simulink model "top_model"  (R2018a)
settings: Solver=FixedStepAuto  StartTime=0.0  StopTime=600  FixedStep=.01  RelTol=1e-3  EnableMultiTasking=on
model workspace: external: MAT-File C:\Users\Justin\Documents\00 MEng Project\PAN_ADCS\initialization\simulink_workspace_init.mat (data not in the file)
undefined symbols (not defined in the file or in its folder): h_init, hdmax, hmax, IAU, Imp_max, Imp_min, init, K_F, Kd, km, Kp, L_F, m_follower, match_tol, muE, ontime_max, ontime_min, q_init, s, Thrust_max, Thrust_min, wbn_init
libraries: aerolibtransform2 x9, hEemethod x8, aerolibconvert2 x6, aerolibgravity2 x5, sharedtransform x4, aerolibutil x4, aerolibcelestial x3, vrlib x2
(part 2 of 3)

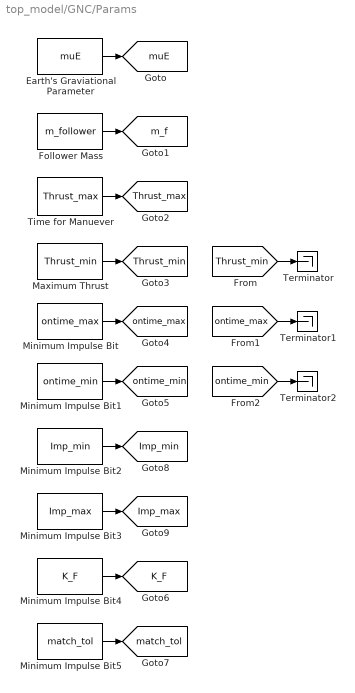
== system top_model/GNC/Params ==
  Earth's Graviational Parameter : Constant  Value=muE
  Follower Mass : Constant  Value=m_follower
  Maximum Thrust : Constant  Value=Thrust_min
  Minimum Impulse Bit : Constant  Value=ontime_max
  Minimum Impulse Bit1 : Constant  Value=ontime_min
  Minimum Impulse Bit2 : Constant  Value=Imp_min
  Minimum Impulse Bit3 : Constant  Value=Imp_max
  Minimum Impulse Bit4 : Constant  Value=K_F
  Minimum Impulse Bit5 : Constant  Value=match_tol
  Terminator : Terminator
  Terminator1 : Terminator
  Terminator2 : Terminator
  Time for Manuever : Constant  Value=Thrust_max
  tag scope: Imp_max=global, Imp_min=global, K_F=global, Thrust_max=global, Thrust_min=global, m_f=global, match_tol=global, muE=global, ontime_max=global, ontime_min=global
  wires:
  Time for Manuever/1 -> [Thrust_max]
  Follower Mass/1 -> [m_f]
  Earth's Graviational Parameter/1 -> [muE]
  Maximum Thrust/1 -> [Thrust_min]
  Minimum Impulse Bit/1 -> [ontime_max]
  Minimum Impulse Bit1/1 -> [ontime_min]
  Minimum Impulse Bit2/1 -> [Imp_min]
  Minimum Impulse Bit3/1 -> [Imp_max]
  [Thrust_min] -> Terminator/1
  [ontime_max] -> Terminator1/1
  [ontime_min] -> Terminator2/1
  Minimum Impulse Bit4/1 -> [K_F]
  Minimum Impulse Bit5/1 -> [match_tol]

== system top_model/LDR_Plant/Cross ==
  A : Inport
  B : Inport  Port=2
  Mux4 : Mux  Inputs=3
  Product{,1..5} (6 alike) : Product  SaturateOnIntegerOverflow=on  InputSameDT=on  OutDataTypeStr=Inherit: Same as first input
  Sum : Sum  Inputs=+-  SaturateOnIntegerOverflow=on  InputSameDT=on  OutDataTypeStr=Inherit: Same as first input
  Sum1 : Sum  Inputs=+-  SaturateOnIntegerOverflow=on  InputSameDT=on  OutDataTypeStr=Inherit: Same as first input
  Sum2 : Sum  Inputs=+-  SaturateOnIntegerOverflow=on  InputSameDT=on  OutDataTypeStr=Inherit: Same as first input
  demux2 : Demux  Outputs=3
  demux3 : Demux  Outputs=3
  AxB : Outport  InitialOutput=0
  wires:
  Mux4/1 -> AxB/1
  Sum2/1 -> Mux4/3
  Sum1/1 -> Mux4/2
  Sum/1 -> Mux4/1
  Product5/1 -> Sum2/2
  Product4/1 -> Sum2/1
  Product3/1 -> Sum1/2
  Product2/1 -> Sum1/1
  Product1/1 -> Sum/2
  Product/1 -> Sum/1
  demux3/1 -> Product5/2, Product2/2
  demux2/2 -> Product5/1, Product/1
  demux3/2 -> Product4/2, Product1/2
  demux2/1 -> Product4/1, Product3/1
  demux3/3 -> Product3/2, Product/2
  demux2/3 -> Product2/1, Product1/1
  B/1 -> demux3/1
  A/1 -> demux2/1

== system top_model/LDR_Plant/DecimalYearIncrement ==
  note: day
  clock_sec : Inport
  Add : Sum
  Constant : Constant  Value=init.year
  Constant1 : Constant  Value=init.month
  Constant2 : Constant  Value=init.day
  Constant3 : Constant  Value=init.hour
  Constant4 : Constant  Value=init.min
  Constant5 : Constant  Value=init.min
  Divide : Product  Inputs=*/
  MATLAB Function : MATLAB Function  TreatAsAtomicUnit=on
  Product2 : Product  Inputs=*/
  day2decimalYear : Constant  Value=365
  sec2day : Constant  Value=86400
  DecimalYear : Outport
  wires:
  Product2/1 -> Divide/1
  sec2day/1 -> Product2/2
  Add/1 -> DecimalYear/1
  Constant3/1 -> MATLAB Function/4(hour)
  day2decimalYear/1 -> Divide/2
  Divide/1 -> Add/1
  MATLAB Function/1(DecimalYear) -> Add/2
  Constant1/1 -> MATLAB Function/2(month)
  Constant/1 -> MATLAB Function/1(year)
  Constant4/1 -> MATLAB Function/5(minute)
  Constant5/1 -> MATLAB Function/6(second)
  clock_sec/1 -> Product2/1
  Constant2/1 -> MATLAB Function/3(day)

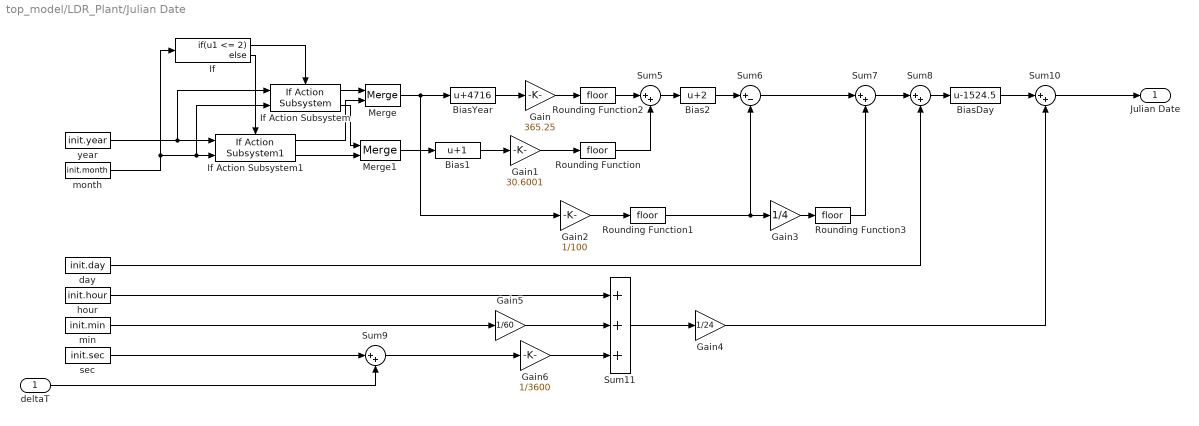
== system top_model/LDR_Plant/Julian Date ==
  deltaT : Inport  OutMin=0  PortDimensions=1
  Bias1 : Bias  Bias=1
  Bias2 : Bias  Bias=2
  BiasDay : Bias  Bias=-1524.5
  BiasYear : Bias  Bias=4716
  Gain : Gain  Gain=365.25
  Gain1 : Gain  Gain=30.6001
  Gain2 : Gain  Gain=1/100
  Gain3 : Gain  Gain=1/4
  Gain4 : Gain  Gain=1/24
  Gain5 : Gain  Gain=1/60
  Gain6 : Gain  Gain=1/3600
  If : If  IfExpression=u1 <= 2
  If Action Subsystem : aerolibconvert2/Julian Date Conversion/If Action Subsystem
      settings: SourceProductName=Aerospace Blockset  SourceProductBaseCode=AE
  If Action Subsystem1 : aerolibconvert2/Julian Date Conversion/If Action Subsystem1
      settings: SourceProductName=Aerospace Blockset  SourceProductBaseCode=AE
  Merge : Merge
  Merge1 : Merge
  Rounding Function{,1..3} (4 alike) : Rounding
  Sum{5,7..10} (5 alike) : Sum  Inputs=|++
  Sum11 : Sum  Inputs=+++
  Sum6 : Sum  Inputs=|+-
  day : Constant  Value=init.day
  hour : Constant  Value=init.hour
  min : Constant  Value=init.min
  month : Constant  Value=init.month
  sec : Constant  Value=init.sec
  year : Constant  Value=init.year
  Julian Date : Outport
  wires:
  If Action Subsystem/1 -> Merge/1
  If/2 -> If Action Subsystem1/Action
  year/1 -> If Action Subsystem/1, If Action Subsystem1/1
  If/1 -> If Action Subsystem/Action
  If Action Subsystem/2 -> Merge1/1
  Rounding Function3/1 -> Sum7/2
  deltaT/1 -> Sum9/2
  Merge1/1 -> Bias1/1
  Gain/1 -> Rounding Function2/1
  Gain2/1 -> Rounding Function1/1
  Merge/1 -> Gain2/1, BiasYear/1
  Sum9/1 -> Gain6/1
  Sum6/1 -> Sum7/1
  Gain5/1 -> Sum11/2
  BiasYear/1 -> Gain/1
  min/1 -> Gain5/1
  Gain6/1 -> Sum11/3
  Sum11/1 -> Gain4/1
  Gain3/1 -> Rounding Function3/1
  hour/1 -> Sum11/1
  If Action Subsystem1/1 -> Merge/2
  Sum7/1 -> Sum8/1
  Sum10/1 -> Julian Date/1
  day/1 -> Sum8/2
  Bias1/1 -> Gain1/1
  sec/1 -> Sum9/1
  If Action Subsystem1/2 -> Merge1/2
  Sum5/1 -> Bias2/1
  BiasDay/1 -> Sum10/1
  Gain1/1 -> Rounding Function/1
  Rounding Function1/1 -> Gain3/1, Sum6/2
  Bias2/1 -> Sum6/1
  Sum8/1 -> BiasDay/1
  Rounding Function2/1 -> Sum5/1
  Rounding Function/1 -> Sum5/2
  month/1 -> If Action Subsystem/2, If Action Subsystem1/2, If/1
  Gain4/1 -> Sum10/2

== system top_model/LDR_Plant/Quaternion Integration ==
  w_Body : Inport
  Gain : Gain  Gain=-1
  Integrator1 : Integrator  InitialCondition=init.LDR.q_init  ContinuousStateAttributes='quaternion_plant'
  Selector : Selector  InputPortWidth=4  IndexOptions=Index vector (dialog)  Indices=4  OutputSizes=1
  Switch : Switch  Criteria=u2 > Threshold
  q_normalize : Subsystem
  qderiv : Subsystem
  q_I_Body : Outport
  wires:
  qderiv/1(qd) -> Integrator1/1
  Integrator1/1 -> q_normalize/1(q_in)
  q_normalize/1(q_out) -> Gain/1, Selector/1, q_I_Body/1, Switch/1, qderiv/2(q)
  w_Body/1 -> qderiv/1(w)
  Selector/1 -> Switch/2
  Gain/1 -> Switch/3

== system top_model/LDR_Sensor Model/Magnetometer ==
  note: Magnetometer: LIS3MDL
      | see the data sheet for more details
  Magnetic_Field_body : Inport  Unit=nT
  DCM to translate from body to sensor : Constant  Value=init.IMU0_DCM_BODY
  Data Type Conversion : DataTypeConversion  OutDataTypeStr=int16  RndMeth=Round
  Matrix Multiply2 : Product  Multiplication=Matrix(*)
  Random Number : RandomNumber  Mean=-init.IMU0_ZGAUSS  Variance=init.IMU0_RMS^2  SampleTime=1.0/init.IMU0_MAG_ODR
  Sum : Sum  Inputs=|++
  Zero-Order Hold : ZeroOrderHold  SampleTime=1.0/init.IMU0_MAG_ODR
  nT to gauss : Gain  Gain=1.0e-5
  sensitivity : Gain  Gain=init.IMU0_MAG_GN
  Magxyz : Outport  OutDataTypeStr=int16
  wires:
  Data Type Conversion/1 -> Magxyz/1
  sensitivity/1 -> Data Type Conversion/1
  nT to gauss/1 -> Zero-Order Hold/1
  Zero-Order Hold/1 -> Sum/1
  Sum/1 -> sensitivity/1
  Random Number/1 -> Sum/2
  Matrix Multiply2/1 -> nT to gauss/1
  Magnetic_Field_body/1 -> Matrix Multiply2/2
  DCM to translate from body to sensor/1 -> Matrix Multiply2/1

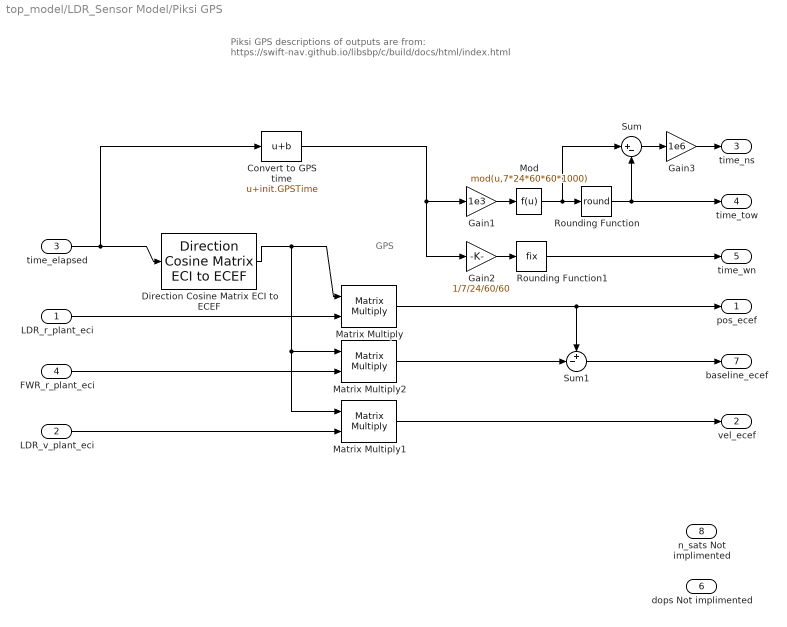
== system top_model/LDR_Sensor Model/Piksi GPS ==
  note: Piksi GPS
      |
      | descriptions of outputs are from:
      | https://swift-nav.github.io/libsbp/c/build/docs/html/index.html
  note: GPS
  LDR_r_plant_eci : Inport
  LDR_v_plant_eci : Inport  Port=2
  time_elapsed : Inport  Port=3
  FWR_r_plant_eci : Inport  Port=4
  Convert to GPS time : Bias  Bias=init.GPSTime
  Direction Cosine Matrix ECI to ECEF : aerolibtransform2/Direction Cosine Matrix ECI to ECEF  red=IAU-2000/2006  year=init.year  month=October  day=20  hour=init.hour  min=init.min  sec=init.sec  deltaT=Sec  errorflag=Error  extraparamflag=off
      settings: AttributesFormatString=%<red>  SourceProductName=Aerospace Blockset  SourceProductBaseCode=AE
  Gain1 : Gain  Gain=1e3
  Gain2 : Gain  Gain=1/7/24/60/60
  Gain3 : Gain  Gain=1e6
  Matrix Multiply : Product  Multiplication=Matrix(*)
  Matrix Multiply1 : Product  Multiplication=Matrix(*)
  Matrix Multiply2 : Product  Multiplication=Matrix(*)
  Mod : Fcn  Expr=mod(u,7*24*60*60*1000)
  Rounding Function : Rounding  Operator=round
  Rounding Function1 : Rounding  Operator=fix
  Sum : Sum  Inputs=|+-
  Sum1 : Sum  Inputs=+-|
  pos_ecef : Outport  OutDataTypeStr=double  Unit=m
      settings: AttributesFormatString=absolute Earth Centered Earth Fixed (ECEF) coordinates
  vel_ecef : Outport  Port=2  OutDataTypeStr=int32  Unit=mm/s
      settings: AttributesFormatString=velocity in Earth Centered Earth Fixed (ECEF) coordinates.
  time_ns : Outport  Port=3  OutMin=[-500000]  OutMax=[500000]  OutDataTypeStr=int32  Unit=ns
      settings: AttributesFormatString=Nanosecond residual of millisecond-rounded TOW
  time_tow : Outport  Port=4  OutMin=[0]  OutDataTypeStr=uint32  Unit=ms
      settings: AttributesFormatString=GPS time of week rounded to the nearest millisecond
  time_wn : Outport  Port=5  OutDataTypeStr=uint16  Unit=weeks
      settings: AttributesFormatString=GPS week number
  dops Not implimented : Outport  Port=6
      settings: AttributesFormatString=|
      | Dilution of Precision p,t
      | describes the effect of navigation satellite geometry on positional measurement precision.
  baseline_ecef : Outport  Description=Dilution of Precision p,t  Port=7  OutDataTypeStr=int32  Unit=mm
      settings: AttributesFormatString=relative vector distance from the base station to the rover receiver.
  n_sats Not implimented : Outport  Port=8  OutDataTypeStr=uint8
      settings: AttributesFormatString=Number of satellites used in solution.
  wires:
  Direction Cosine Matrix ECI to ECEF/1 -> Matrix Multiply1/1, Matrix Multiply2/1, Matrix Multiply/1
  time_elapsed/1 -> Convert to GPS time/1, Direction Cosine Matrix ECI to ECEF/1
  LDR_v_plant_eci/1 -> Matrix Multiply1/2
  Matrix Multiply1/1 -> vel_ecef/1
  Matrix Multiply/1 -> Sum1/1, pos_ecef/1
  LDR_r_plant_eci/1 -> Matrix Multiply/2
  Convert to GPS time/1 -> Gain2/1, Gain1/1
  Gain2/1 -> Rounding Function1/1
  Rounding Function1/1 -> time_wn/1
  Gain1/1 -> Mod/1
  Mod/1 -> Sum/1, Rounding Function/1
  Rounding Function/1 -> Sum/2, time_tow/1
  Sum/1 -> Gain3/1
  Gain3/1 -> time_ns/1
  FWR_r_plant_eci/1 -> Matrix Multiply2/2
  Sum1/1 -> baseline_ecef/1
  Matrix Multiply2/1 -> Sum1/2

== system top_model/LDR_Sensor Model/quat to DCM ==
  e0 e1 e2 e3 : Inport
  Demux : Demux
  Gain1 : Gain  Gain=2  SaturateOnIntegerOverflow=on  OutDataTypeStr=Inherit: Same as input  ParamDataTypeStr=Inherit: Same as input
  Gain2 : Gain  Gain=2  SaturateOnIntegerOverflow=on  OutDataTypeStr=Inherit: Same as input  ParamDataTypeStr=Inherit: Same as input
  Matrix Gain : Gain  Gain=eye(3,3)  SaturateOnIntegerOverflow=on  OutDataTypeStr=Inherit: Same as input  ParamDataTypeStr=Inherit: Same as input
  Mux : Mux  Inputs=3
  Product : Product  SaturateOnIntegerOverflow=on  InputSameDT=on  OutDataTypeStr=Inherit: Same as first input
  Product1 : Product  SaturateOnIntegerOverflow=on  InputSameDT=on  OutDataTypeStr=Inherit: Same as first input
  Subsystem : Subsystem
      mask Display: disp('3x3 cross matrix')
  Sum1 : Sum  Inputs=|+-  SaturateOnIntegerOverflow=on  InputSameDT=on  OutDataTypeStr=Inherit: Same as first input
  Sum8 : Sum  Inputs=|+-+  SaturateOnIntegerOverflow=on  InputSameDT=on  OutDataTypeStr=Inherit: Same as first input
  T1 : Math  Operator=transpose  SaturateOnIntegerOverflow=on
  T2 : Math  Operator=transpose  SaturateOnIntegerOverflow=on
  qTq : Product  Multiplication=Matrix(*)  SaturateOnIntegerOverflow=on  InputSameDT=on  OutDataTypeStr=Inherit: Same as first input
  qqT : Product  Multiplication=Matrix(*)  SaturateOnIntegerOverflow=on  InputSameDT=on  OutDataTypeStr=Inherit: Same as first input
  DCM : Outport  InitialOutput=0
  wires:
  Sum8/1 -> DCM/1
  e0 e1 e2 e3/1 -> Demux/1
  Demux/1 -> Mux/1
  Demux/2 -> Mux/2
  Demux/3 -> Mux/3
  Demux/4 -> Product/2, Product1/1, Product1/2
  Mux/1 -> T1/1, qqT/1, Subsystem/1(In1), T2/1, qTq/2
  Product/1 -> Gain1/1
  T1/1 -> qqT/2
  qqT/1 -> Gain2/1
  Gain2/1 -> Sum8/1
  Gain1/1 -> Sum8/2
  Product1/1 -> Sum1/1
  T2/1 -> qTq/1
  qTq/1 -> Sum1/2
  Sum1/1 -> Matrix Gain/1
  Matrix Gain/1 -> Sum8/3
  Subsystem/1(Out1) -> Product/1

== system top_model/Actuator Model/Rigid Body with Momentum Actuators and energy dissipation/Cross1 ==
  A : Inport  PortDimensions=3
  B : Inport  Port=2  PortDimensions=3
  Mux4 : Mux  Inputs=3
  Product{,1..5} (6 alike) : Product  SaturateOnIntegerOverflow=on  InputSameDT=on  OutDataTypeStr=Inherit: Same as first input
  Sum : Sum  Inputs=+-  SaturateOnIntegerOverflow=on  InputSameDT=on  OutDataTypeStr=Inherit: Same as first input
  Sum1 : Sum  Inputs=+-  SaturateOnIntegerOverflow=on  InputSameDT=on  OutDataTypeStr=Inherit: Same as first input
  Sum2 : Sum  Inputs=+-  SaturateOnIntegerOverflow=on  InputSameDT=on  OutDataTypeStr=Inherit: Same as first input
  demux2 : Demux  Outputs=3
  demux3 : Demux  Outputs=3
  AxB : Outport  InitialOutput=0
  wires:
  Mux4/1 -> AxB/1
  Sum2/1 -> Mux4/3
  Sum1/1 -> Mux4/2
  Sum/1 -> Mux4/1
  Product5/1 -> Sum2/2
  Product4/1 -> Sum2/1
  Product3/1 -> Sum1/2
  Product2/1 -> Sum1/1
  Product1/1 -> Sum/2
  Product/1 -> Sum/1
  demux3/1 -> Product5/2, Product2/2
  demux2/2 -> Product5/1, Product/1
  demux3/2 -> Product4/2, Product1/2
  demux2/1 -> Product4/1, Product3/1
  demux3/3 -> Product3/2, Product/2
  demux2/3 -> Product2/1, Product1/1
  B/1 -> demux3/1
  A/1 -> demux2/1

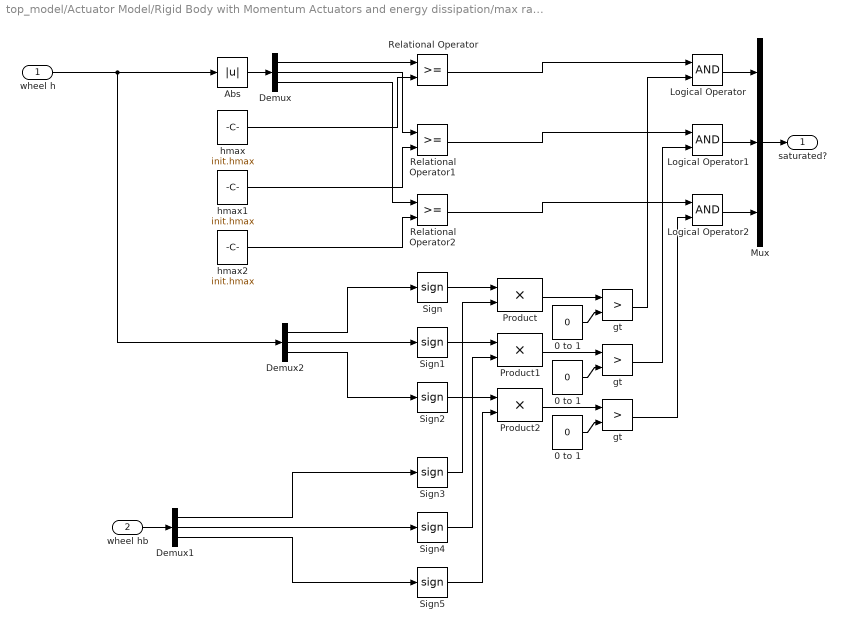
== system top_model/Actuator Model/Rigid Body with Momentum Actuators and energy dissipation/max rate check ==
  wheel h : Inport
  wheel hb : Inport  Port=2
  0 to 1 : Constant  Value=0  VectorParams1D=off
  "0 to 1 " : Constant  Value=0  VectorParams1D=off
  "0 to 1  " : Constant  Value=0  VectorParams1D=off
  Abs : Abs  SaturateOnIntegerOverflow=on
  Demux : Demux  Outputs=3
  Demux1 : Demux  Outputs=3
  Demux2 : Demux  Outputs=3
  Logical Operator : Logic
  Logical Operator1 : Logic
  Logical Operator2 : Logic
  Mux : Mux  Inputs=3
  Product : Product  SaturateOnIntegerOverflow=on  InputSameDT=on  OutDataTypeStr=Inherit: Same as first input
  Product1 : Product  SaturateOnIntegerOverflow=on  InputSameDT=on  OutDataTypeStr=Inherit: Same as first input
  Product2 : Product  SaturateOnIntegerOverflow=on  InputSameDT=on  OutDataTypeStr=Inherit: Same as first input
  Relational Operator : RelationalOperator  RndMeth=Nearest  InputSameDT=on
  Relational Operator1 : RelationalOperator  RndMeth=Nearest  InputSameDT=on
  Relational Operator2 : RelationalOperator  RndMeth=Nearest  InputSameDT=on
  Sign{,1..5} (6 alike) : Signum
  gt : RelationalOperator  Operator=>  RndMeth=Nearest  InputSameDT=on
  "gt " : RelationalOperator  Operator=>  RndMeth=Nearest  InputSameDT=on
  "gt  " : RelationalOperator  Operator=>  RndMeth=Nearest  InputSameDT=on
  hmax : Constant  Value=init.hmax  VectorParams1D=off
  hmax1 : Constant  Value=init.hmax  VectorParams1D=off
  hmax2 : Constant  Value=init.hmax  VectorParams1D=off
  saturated? : Outport
  wires:
  Abs/1 -> Demux/1
  Demux/1 -> Relational Operator/1
  Demux/2 -> Relational Operator1/1
  Demux/3 -> Relational Operator2/1
  hmax/1 -> Relational Operator/2
  hmax1/1 -> Relational Operator1/2
  hmax2/1 -> Relational Operator2/2
  wheel h/1 -> Abs/1, Demux2/1
  Mux/1 -> saturated?/1
  wheel hb/1 -> Demux1/1
  Demux1/1 -> Sign3/1
  Demux1/2 -> Sign4/1
  Demux1/3 -> Sign5/1
  Sign/1 -> Product/1
  Sign3/1 -> Product/2
  Sign1/1 -> Product1/1
  Sign4/1 -> Product1/2
  Sign2/1 -> Product2/1
  Sign5/1 -> Product2/2
  0 to 1/1 -> gt/2
  Product/1 -> gt/1
  "0 to 1 "/1 -> "gt "/2
  Product1/1 -> "gt "/1
  "0 to 1  "/1 -> "gt  "/2
  Product2/1 -> "gt  "/1
  Logical Operator/1 -> Mux/1
  Logical Operator1/1 -> Mux/2
  Logical Operator2/1 -> Mux/3
  Relational Operator/1 -> Logical Operator/1
  Relational Operator1/1 -> Logical Operator1/1
  Relational Operator2/1 -> Logical Operator2/1
  gt/1 -> Logical Operator/2
  "gt "/1 -> Logical Operator1/2
  "gt  "/1 -> Logical Operator2/2
  Demux2/1 -> Sign/1
  Demux2/2 -> Sign1/1
  Demux2/3 -> Sign2/1

== system top_model/Actuator Model/Rigid Body with Momentum Actuators and energy dissipation/quat to DCM ==
  e0 e1 e2 e3 : Inport
  Demux : Demux
  Gain1 : Gain  Gain=2  SaturateOnIntegerOverflow=on  OutDataTypeStr=Inherit: Same as input  ParamDataTypeStr=Inherit: Same as input
  Gain2 : Gain  Gain=2  SaturateOnIntegerOverflow=on  OutDataTypeStr=Inherit: Same as input  ParamDataTypeStr=Inherit: Same as input
  Matrix Gain : Gain  Gain=eye(3,3)  SaturateOnIntegerOverflow=on  OutDataTypeStr=Inherit: Same as input  ParamDataTypeStr=Inherit: Same as input
  Mux : Mux  Inputs=3
  Product : Product  SaturateOnIntegerOverflow=on  InputSameDT=on  OutDataTypeStr=Inherit: Same as first input
  Product1 : Product  SaturateOnIntegerOverflow=on  InputSameDT=on  OutDataTypeStr=Inherit: Same as first input
  Subsystem : Subsystem
      mask Display: disp('3x3 cross matrix')
  Sum1 : Sum  Inputs=|+-  SaturateOnIntegerOverflow=on  InputSameDT=on  OutDataTypeStr=Inherit: Same as first input
  Sum8 : Sum  Inputs=|+-+  SaturateOnIntegerOverflow=on  InputSameDT=on  OutDataTypeStr=Inherit: Same as first input
  T1 : Math  Operator=transpose  SaturateOnIntegerOverflow=on
  T2 : Math  Operator=transpose  SaturateOnIntegerOverflow=on
  qTq : Product  Multiplication=Matrix(*)  SaturateOnIntegerOverflow=on  InputSameDT=on  OutDataTypeStr=Inherit: Same as first input
  qqT : Product  Multiplication=Matrix(*)  SaturateOnIntegerOverflow=on  InputSameDT=on  OutDataTypeStr=Inherit: Same as first input
  DCM : Outport  InitialOutput=0
  wires:
  Subsystem/1(Out1) -> Product/1
  Matrix Gain/1 -> Sum8/3
  Sum1/1 -> Matrix Gain/1
  qTq/1 -> Sum1/2
  T2/1 -> qTq/1
  Product1/1 -> Sum1/1
  Gain1/1 -> Sum8/2
  Gain2/1 -> Sum8/1
  qqT/1 -> Gain2/1
  T1/1 -> qqT/2
  Product/1 -> Gain1/1
  Mux/1 -> qTq/2, T2/1, qqT/1, T1/1, Subsystem/1(In1)
  Demux/4 -> Product1/2, Product1/1, Product/2
  Demux/3 -> Mux/3
  Demux/2 -> Mux/2
  Demux/1 -> Mux/1
  e0 e1 e2 e3/1 -> Demux/1
  Sum8/1 -> DCM/1

== system top_model/Actuator Model/Rigid Body with Momentum Actuators and energy dissipation/quat to DCM1 ==
  e0 e1 e2 e3 : Inport
  Demux : Demux
  Gain1 : Gain  Gain=2  SaturateOnIntegerOverflow=on  OutDataTypeStr=Inherit: Same as input  ParamDataTypeStr=Inherit: Same as input
  Gain2 : Gain  Gain=2  SaturateOnIntegerOverflow=on  OutDataTypeStr=Inherit: Same as input  ParamDataTypeStr=Inherit: Same as input
  Matrix Gain : Gain  Gain=eye(3,3)  SaturateOnIntegerOverflow=on  OutDataTypeStr=Inherit: Same as input  ParamDataTypeStr=Inherit: Same as input
  Mux : Mux  Inputs=3
  Product : Product  SaturateOnIntegerOverflow=on  InputSameDT=on  OutDataTypeStr=Inherit: Same as first input
  Product1 : Product  SaturateOnIntegerOverflow=on  InputSameDT=on  OutDataTypeStr=Inherit: Same as first input
  Subsystem : Subsystem
      mask Display: disp('3x3 cross matrix')
  Sum1 : Sum  Inputs=|+-  SaturateOnIntegerOverflow=on  InputSameDT=on  OutDataTypeStr=Inherit: Same as first input
  Sum8 : Sum  Inputs=|+-+  SaturateOnIntegerOverflow=on  InputSameDT=on  OutDataTypeStr=Inherit: Same as first input
  T1 : Math  Operator=transpose  SaturateOnIntegerOverflow=on
  T2 : Math  Operator=transpose  SaturateOnIntegerOverflow=on
  qTq : Product  Multiplication=Matrix(*)  SaturateOnIntegerOverflow=on  InputSameDT=on  OutDataTypeStr=Inherit: Same as first input
  qqT : Product  Multiplication=Matrix(*)  SaturateOnIntegerOverflow=on  InputSameDT=on  OutDataTypeStr=Inherit: Same as first input
  DCM : Outport  InitialOutput=0
  wires:
  Subsystem/1(Out1) -> Product/1
  Matrix Gain/1 -> Sum8/3
  Sum1/1 -> Matrix Gain/1
  qTq/1 -> Sum1/2
  T2/1 -> qTq/1
  Product1/1 -> Sum1/1
  Gain1/1 -> Sum8/2
  Gain2/1 -> Sum8/1
  qqT/1 -> Gain2/1
  T1/1 -> qqT/2
  Product/1 -> Gain1/1
  Mux/1 -> qTq/2, T2/1, qqT/1, T1/1, Subsystem/1(In1)
  Demux/4 -> Product1/2, Product1/1, Product/2
  Demux/3 -> Mux/3
  Demux/2 -> Mux/2
  Demux/1 -> Mux/1
  e0 e1 e2 e3/1 -> Demux/1
  Sum8/1 -> DCM/1

== system top_model/Attitude Determination and Desired Attitude/Attitude Determination/Generate reference vectors from Ephemeris and Magnetic Field Model ==
  note: geodetic LLA
  time_elapsed : Inport
  r_cs_sensor_eci : Inport  Port=2
  Add : Sum  Inputs=+-
  DecimalYearIncrement : Subsystem
  Demux : Demux  Outputs=3
  ECI Position to LLA : aerolibtransform2/ECI Position to LLA  red=IAU-2000/2006  year=init.year  month=October  day=20  hour=init.hour  min=init.min  sec=init.sec  deltaT=Sec  errorflag=Error  extraparamflag=off  eunits=Metric (MKS)  earthmodel=WGS84  flat=1/298.257223563  eqradius=6378137
      settings: AttributesFormatString=%<red>  SourceProductName=Aerospace Blockset  SourceProductBaseCode=AE
  International Geomagnetic Reference Field 12 : aerolibgravity2/International Geomagnetic Reference Field 12  units=Metric (MKS)  time_in=on  month=January  day=1  year=2020  action=None  sv_out=off
      settings: SourceProductName=Aerospace Blockset  SourceProductBaseCode=AE
  Julian Date : Subsystem
  Planetary Ephemeris : aerolibcelestial/Planetary Ephemeris  kmflag=km,km/s  epochflag=Julian date  de=DE430  nCenter=Earth  nTarget=Sun  errorflag=Error  velflag=off
      settings: SourceProductName=Aerospace Blockset  SourceProductBaseCode=AE
  r_Sun2cs_ref_eci : Outport
  r_MagField_ref_eci : Outport  Port=2
  wires:
  Julian Date/1(Julian Date) -> Planetary Ephemeris/1
  Planetary Ephemeris/1 -> Add/1
  Demux/1 -> International Geomagnetic Reference Field 12/2
  International Geomagnetic Reference Field 12/1 -> r_MagField_ref_eci/1
  ECI Position to LLA/1 -> Demux/1
  Demux/3 -> International Geomagnetic Reference Field 12/1
  Add/1 -> r_Sun2cs_ref_eci/1
  DecimalYearIncrement/1(DecimalYear) -> International Geomagnetic Reference Field 12/4
  r_cs_sensor_eci/1 -> Add/2, ECI Position to LLA/1
  time_elapsed/1 -> DecimalYearIncrement/1(clock_sec), ECI Position to LLA/2, Julian Date/1(deltaT)
  Demux/2 -> International Geomagnetic Reference Field 12/3

== system top_model/Attitude Determination and Desired Attitude/Attitude Determination/Subsystem ==
  r_Sun2cs_ref_eci : Inport
  r_MagField_ref_eci : Inport  Port=2
  r_Sun2cs_sensor_body : Inport  Port=3
  r_MagField_sensor_body : Inport  Port=4
  MATLAB Function : MATLAB Function  TreatAsAtomicUnit=on
  quat_body_calc : Outport
  wires:
  r_Sun2cs_ref_eci/1 -> MATLAB Function/1(N_sun)
  r_MagField_ref_eci/1 -> MATLAB Function/2(N_mag)
  r_Sun2cs_sensor_body/1 -> MATLAB Function/3(B_sun)
  r_MagField_sensor_body/1 -> MATLAB Function/4(B_mag)
  MATLAB Function/1(q_triad) -> quat_body_calc/1

== system top_model/Attitude Determination and Desired Attitude/Position and Velocity to Desired Attitude in Quat/CreateDCM_be ==
  Position : Inport
  Velocity : Inport  Port=2
  Cross Product : vrlib/Utilities/Cross Product
      settings: SourceProductBaseCode=VR
  Cross Product1 : vrlib/Utilities/Cross Product
      settings: SourceProductBaseCode=VR
  Matrix Concatenate : Concatenate  NumInputs=3  Mode=Multidimensional array  ConcatenateDimension=2
  normalize : Subsystem
  normalize2 : Subsystem
  DCM_be : Outport
  wires:
  normalize/1(r_hat) -> Cross Product1/1, Matrix Concatenate/1
  Cross Product/1 -> normalize2/1(v)
  Velocity/1 -> Cross Product/1
  Matrix Concatenate/1 -> DCM_be/1
  Position/1 -> Cross Product/2, normalize/1(r)
  Cross Product1/1 -> Matrix Concatenate/3
  normalize2/1(v_hat) -> Cross Product1/2, Matrix Concatenate/2

== system top_model/Attitude Determination and Desired Attitude/Position and Velocity to Desired Attitude in Quat/quat to DCM ==
  e0 e1 e2 e3 : Inport
  Demux : Demux
  Gain1 : Gain  Gain=2  SaturateOnIntegerOverflow=on  OutDataTypeStr=Inherit: Same as input  ParamDataTypeStr=Inherit: Same as input
  Gain2 : Gain  Gain=2  SaturateOnIntegerOverflow=on  OutDataTypeStr=Inherit: Same as input  ParamDataTypeStr=Inherit: Same as input
  Matrix Gain : Gain  Gain=eye(3,3)  SaturateOnIntegerOverflow=on  OutDataTypeStr=Inherit: Same as input  ParamDataTypeStr=Inherit: Same as input
  Mux : Mux  Inputs=3
  Product : Product  SaturateOnIntegerOverflow=on  InputSameDT=on  OutDataTypeStr=Inherit: Same as first input
  Product1 : Product  SaturateOnIntegerOverflow=on  InputSameDT=on  OutDataTypeStr=Inherit: Same as first input
  Subsystem : Subsystem
      mask Display: disp('3x3 cross matrix')
  Sum1 : Sum  Inputs=|+-  SaturateOnIntegerOverflow=on  InputSameDT=on  OutDataTypeStr=Inherit: Same as first input
  Sum8 : Sum  Inputs=|+-+  SaturateOnIntegerOverflow=on  InputSameDT=on  OutDataTypeStr=Inherit: Same as first input
  T1 : Math  Operator=transpose  SaturateOnIntegerOverflow=on
  T2 : Math  Operator=transpose  SaturateOnIntegerOverflow=on
  qTq : Product  Multiplication=Matrix(*)  SaturateOnIntegerOverflow=on  InputSameDT=on  OutDataTypeStr=Inherit: Same as first input
  qqT : Product  Multiplication=Matrix(*)  SaturateOnIntegerOverflow=on  InputSameDT=on  OutDataTypeStr=Inherit: Same as first input
  DCM : Outport  InitialOutput=0
  wires:
  Subsystem/1(Out1) -> Product/1
  Matrix Gain/1 -> Sum8/3
  Sum1/1 -> Matrix Gain/1
  qTq/1 -> Sum1/2
  T2/1 -> qTq/1
  Product1/1 -> Sum1/1
  Gain1/1 -> Sum8/2
  Gain2/1 -> Sum8/1
  qqT/1 -> Gain2/1
  T1/1 -> qqT/2
  Product/1 -> Gain1/1
  Mux/1 -> qTq/2, T2/1, qqT/1, T1/1, Subsystem/1(In1)
  Demux/4 -> Product1/2, Product1/1, Product/2
  Demux/3 -> Mux/3
  Demux/2 -> Mux/2
  Demux/1 -> Mux/1
  e0 e1 e2 e3/1 -> Demux/1
  Sum8/1 -> DCM/1

== system top_model/Controller/Free Rigid Body with Momentum Actuators2/Cross ==
  A : Inport
  B : Inport  Port=2
  Mux4 : Mux  Inputs=3
  Product{,1..5} (6 alike) : Product  SaturateOnIntegerOverflow=on  InputSameDT=on  OutDataTypeStr=Inherit: Same as first input
  Sum : Sum  Inputs=+-  SaturateOnIntegerOverflow=on  InputSameDT=on  OutDataTypeStr=Inherit: Same as first input
  Sum1 : Sum  Inputs=+-  SaturateOnIntegerOverflow=on  InputSameDT=on  OutDataTypeStr=Inherit: Same as first input
  Sum2 : Sum  Inputs=+-  SaturateOnIntegerOverflow=on  InputSameDT=on  OutDataTypeStr=Inherit: Same as first input
  demux2 : Demux  Outputs=3
  demux3 : Demux  Outputs=3
  AxB : Outport  InitialOutput=0
  wires:
  Mux4/1 -> AxB/1
  Sum2/1 -> Mux4/3
  Sum1/1 -> Mux4/2
  Sum/1 -> Mux4/1
  Product5/1 -> Sum2/2
  Product4/1 -> Sum2/1
  Product3/1 -> Sum1/2
  Product2/1 -> Sum1/1
  Product1/1 -> Sum/2
  Product/1 -> Sum/1
  demux3/1 -> Product5/2, Product2/2
  demux2/2 -> Product5/1, Product/1
  demux3/2 -> Product4/2, Product1/2
  demux2/1 -> Product4/1, Product3/1
  demux3/3 -> Product3/2, Product/2
  demux2/3 -> Product2/1, Product1/1
  B/1 -> demux3/1
  A/1 -> demux2/1

== system top_model/Controller/Free Rigid Body with Momentum Actuators2/Quaternion Integration ==
  w_Body : Inport
  Integrator1 : Integrator  InitialCondition=q_init
  q_normalize : Subsystem
  qderiv : Subsystem
  q_I_Body : Outport
  wires:
  qderiv/1(qd) -> Integrator1/1
  Integrator1/1 -> q_normalize/1(q_in)
  q_normalize/1(q_out) -> q_I_Body/1, qderiv/2(q)
  w_Body/1 -> qderiv/1(w)

== system top_model/Controller/Free Rigid Body with Momentum Actuators2/RWA Saturation Model (Maxon EC 32 Flat 15W 24V) ==
  hb_com : Inport
  Demux : Demux  Outputs=3
  Demux2 : Demux  Outputs=3
  Max Torque : Saturate  UpperLimit=hdmax  LowerLimit=-hdmax
  Mux : Mux  Inputs=3
  Scope : Scope
  Switch : Switch  Threshold=0.5  SaturateOnIntegerOverflow=on  InputSameDT=on
  Switch1 : Switch  Threshold=0.5  SaturateOnIntegerOverflow=on  InputSameDT=on
  Switch2 : Switch  Threshold=0.5  SaturateOnIntegerOverflow=on  InputSameDT=on
  "hb -> h" : Integrator  InitialCondition=h_init
  max rate check : Subsystem
  no torque : Constant  Value=0
  hb_act : Outport
  h_act : Outport  Port=2
  wires:
  Switch2/1 -> Mux/3
  Switch1/1 -> Mux/2
  Demux2/3 -> Switch2/2
  Switch/1 -> Mux/1
  no torque/1 -> Switch/1, Switch1/1, Switch2/1
  Demux2/1 -> Switch/2
  Mux/1 -> Scope/1, hb_act/1, "hb -> h"/1
  hb_com/1 -> Max Torque/1
  Demux2/2 -> Switch1/2
  Demux/2 -> Switch1/3
  Demux/1 -> Switch/3
  "hb -> h"/1 -> h_act/1, max rate check/1(wheel h)
  Max Torque/1 -> Demux/1, max rate check/2(wheel hb)
  Demux/3 -> Switch2/3
  max rate check/1(saturated?) -> Demux2/1

== system top_model/Controller/Free Rigid Body with Momentum Actuators2/compute attitude error ==
  quat : Inport
  quat_cmd : Inport  Port=2
  Demux : Demux
  Mux : Mux  Inputs=3
  Mux1 : Mux  Inputs=2
  quat_multiply (relative quat) : Subsystem
  reverse : Gain  Gain=-1  SaturateOnIntegerOverflow=on  OutDataTypeStr=Inherit: Same as input  ParamDataTypeStr=Inherit: Same as input
  quat error : Outport
  wires:
  quat/1 -> quat_multiply (relative quat)/1(q_bc)
  quat_cmd/1 -> Demux/1
  Demux/1 -> Mux/1
  Demux/2 -> Mux/2
  Demux/3 -> Mux/3
  Demux/4 -> reverse/1
  Mux/1 -> Mux1/1
  Mux1/1 -> quat_multiply (relative quat)/2(q_ab)
  reverse/1 -> Mux1/2
  quat_multiply (relative quat)/1(q_ac) -> quat error/1

== system top_model/Controller/Normal Mode Control System/compute attitude error ==
  quat : Inport
  quat_cmd : Inport  Port=2
  Demux : Demux
  Demux1 : Demux
  Mux : Mux  Inputs=3
  Mux1 : Mux  Inputs=2
  Mux2 : Mux  Inputs=3
  Mux3 : Mux  Inputs=2
  Selector : Selector  InputPortWidth=4  IndexOptions=Index vector (dialog)  Indices=4  OutputSizes=1
  Switch : Switch
  quat_multiply (relative quat) : Subsystem
  quat_multiply (relative quat)1 : Subsystem
  reverse : Gain  Gain=-1  SaturateOnIntegerOverflow=on  OutDataTypeStr=Inherit: Same as input  ParamDataTypeStr=Inherit: Same as input
  reverse1 : Gain  Gain=-1  SaturateOnIntegerOverflow=on  OutDataTypeStr=Inherit: Same as input  ParamDataTypeStr=Inherit: Same as input
  quat error : Outport
  wires:
  Demux/1 -> Mux/1
  Demux/2 -> Mux/2
  Demux/3 -> Mux/3
  Mux/1 -> reverse/1
  Mux1/1 -> quat_multiply (relative quat)/2(q_ab)
  Demux/4 -> Mux1/2
  reverse/1 -> Mux1/1
  Mux3/1 -> quat_multiply (relative quat)1/2(q_ab)
  Demux1/1 -> Mux2/1
  Demux1/2 -> Mux2/2
  Demux1/3 -> Mux2/3
  quat_cmd/1 -> Demux1/1, Demux/1
  Mux2/1 -> Mux3/1
  quat/1 -> quat_multiply (relative quat)1/1(q_bc), quat_multiply (relative quat)/1(q_bc)
  Demux1/4 -> reverse1/1
  reverse1/1 -> Mux3/2
  quat_multiply (relative quat)1/1(q_ac) -> Switch/3
  quat_multiply (relative quat)/1(q_ac) -> Selector/1, Switch/1
  Switch/1 -> quat error/1
  Selector/1 -> Switch/2

== system top_model/FWR_Plant/Quaternion Integration/q_normalize ==
  q_in : Inport  PortDimensions=4
  Dot Product : DotProduct  InputSameDT=on  OutDataTypeStr=Inherit: Inherit via internal rule
  Math Function : Math  Operator=sqrt  SaturateOnIntegerOverflow=on
  Product : Product  Inputs=*/  SaturateOnIntegerOverflow=on  InputSameDT=on  OutDataTypeStr=Inherit: Same as first input
  q_out : Outport
  wires:
  Product/1 -> q_out/1
  Math Function/1 -> Product/2
  Dot Product/1 -> Math Function/1
  q_in/1 -> Product/1, Dot Product/2, Dot Product/1

== system top_model/FWR_Plant/Quaternion Integration/qderiv ==
  w : Inport
  q : Inport  Port=2
  Mux : Mux  Inputs=2
  Mux1 : Mux
  qd1 : Fcn  Expr=(u(7)*u(1)-u(6)*u(2)+u(5)*u(3))/2
  qd2 : Fcn  Expr=(u(6)*u(1)+u(7)*u(2)-u(4)*u(3))/2
  qd3 : Fcn  Expr=(-u(5)*u(1)+u(4)*u(2)+u(7)*u(3))/2
  qd4 : Fcn  Expr=(-u(4)*u(1)-u(5)*u(2)-u(6)*u(3))/2
  qd : Outport
  wires:
  Mux1/1 -> qd/1
  qd4/1 -> Mux1/4
  qd3/1 -> Mux1/3
  qd2/1 -> Mux1/2
  qd1/1 -> Mux1/1
  Mux/1 -> qd2/1, qd1/1, qd4/1, qd3/1
  q/1 -> Mux/2
  w/1 -> Mux/1

== system top_model/GNC/Follower Maneuver/Optimal Latitude Calc ==
  "r " : Inport
  "v " : Inport  Port=2
  muE : Inport  Port=3
  x_tgt : Inport  Port=4
  x_f : Inport  Port=5
  Update Trigger : Inport  Port=6
  Constant : Constant  Value=K_F
  Constant1 : Constant  Value=L_F
  Enabled Subsystem : Subsystem  TreatAsAtomicUnit=on
  dV_opt : Outport
  long_opt : Outport  Port=2
  pos_opt : Outport  Port=3
  wires:
  Enabled Subsystem/2(long_opt) -> long_opt/1
  "r "/1 -> Enabled Subsystem/1(r)
  "v "/1 -> Enabled Subsystem/2(v)
  muE/1 -> Enabled Subsystem/7("muE ")
  x_tgt/1 -> Enabled Subsystem/3(x_tgt)
  x_f/1 -> Enabled Subsystem/4(x_f)
  Constant/1 -> Enabled Subsystem/5(K)
  Constant1/1 -> Enabled Subsystem/6(L)
  Enabled Subsystem/1(dV_opt) -> dV_opt/1
  Enabled Subsystem/3(pos_opt) -> pos_opt/1
  Update Trigger/1 -> Enabled Subsystem/Enable

== system top_model/LDR_Plant/Quaternion Integration/q_normalize ==
  q_in : Inport  PortDimensions=4
  Dot Product : DotProduct  InputSameDT=on  OutDataTypeStr=Inherit: Inherit via internal rule
  Math Function : Math  Operator=sqrt  SaturateOnIntegerOverflow=on
  Product : Product  Inputs=*/  SaturateOnIntegerOverflow=on  InputSameDT=on  OutDataTypeStr=Inherit: Same as first input
  q_out : Outport
  wires:
  q_in/1 -> Dot Product/1, Dot Product/2, Product/1
  Dot Product/1 -> Math Function/1
  Math Function/1 -> Product/2
  Product/1 -> q_out/1

== system top_model/LDR_Plant/Quaternion Integration/qderiv ==
  w : Inport
  q : Inport  Port=2
  Mux : Mux  Inputs=2
  Mux1 : Mux
  qd1 : Fcn  Expr=(u(7)*u(1)-u(6)*u(2)+u(5)*u(3))/2
  qd2 : Fcn  Expr=(u(6)*u(1)+u(7)*u(2)-u(4)*u(3))/2
  qd3 : Fcn  Expr=(-u(5)*u(1)+u(4)*u(2)+u(7)*u(3))/2
  qd4 : Fcn  Expr=(-u(4)*u(1)-u(5)*u(2)-u(6)*u(3))/2
  qd : Outport
  wires:
  w/1 -> Mux/1
  q/1 -> Mux/2
  Mux/1 -> qd3/1, qd4/1, qd1/1, qd2/1
  qd1/1 -> Mux1/1
  qd2/1 -> Mux1/2
  qd3/1 -> Mux1/3
  qd4/1 -> Mux1/4
  Mux1/1 -> qd/1

== system top_model/LDR_Sensor Model/quat to DCM/Subsystem ==
  In1 : Inport
  3x3 : Reshape  OutputDimensionality=Customize  OutputDimensions=[3,3]
  Demux : Demux  Outputs=3
  Gain : Gain  Gain=-1  SaturateOnIntegerOverflow=on  OutDataTypeStr=Inherit: Same as input  ParamDataTypeStr=Inherit: Same as input
  Gain1 : Gain  Gain=-1  SaturateOnIntegerOverflow=on  OutDataTypeStr=Inherit: Same as input  ParamDataTypeStr=Inherit: Same as input
  Gain2 : Gain  Gain=-1  SaturateOnIntegerOverflow=on  OutDataTypeStr=Inherit: Same as input  ParamDataTypeStr=Inherit: Same as input
  Mux : Mux  Inputs=9
  "diag 0 " : Constant  Value=0
  Out1 : Outport
  wires:
  In1/1 -> Demux/1
  3x3/1 -> Out1/1
  "diag 0 "/1 -> Mux/1, Mux/5, Mux/9
  Mux/1 -> 3x3/1
  Demux/3 -> Mux/2, Gain1/1
  Gain/1 -> Mux/3
  Demux/2 -> Gain/1, Mux/7
  Gain1/1 -> Mux/4
  Demux/1 -> Mux/6, Gain2/1
  Gain2/1 -> Mux/8

== system top_model/Actuator Model/Rigid Body with Momentum Actuators and energy dissipation/quat to DCM/Subsystem ==
  In1 : Inport
  3x3 : Reshape  OutputDimensionality=Customize  OutputDimensions=[3,3]
  Demux : Demux  Outputs=3
  Gain : Gain  Gain=-1  SaturateOnIntegerOverflow=on  OutDataTypeStr=Inherit: Same as input  ParamDataTypeStr=Inherit: Same as input
  Gain1 : Gain  Gain=-1  SaturateOnIntegerOverflow=on  OutDataTypeStr=Inherit: Same as input  ParamDataTypeStr=Inherit: Same as input
  Gain2 : Gain  Gain=-1  SaturateOnIntegerOverflow=on  OutDataTypeStr=Inherit: Same as input  ParamDataTypeStr=Inherit: Same as input
  Mux : Mux  Inputs=9
  "diag 0 " : Constant  Value=0
  Out1 : Outport
  wires:
  Gain2/1 -> Mux/8
  Demux/1 -> Gain2/1, Mux/6
  Gain1/1 -> Mux/4
  Demux/2 -> Mux/7, Gain/1
  Gain/1 -> Mux/3
  Demux/3 -> Gain1/1, Mux/2
  Mux/1 -> 3x3/1
  "diag 0 "/1 -> Mux/9, Mux/5, Mux/1
  3x3/1 -> Out1/1
  In1/1 -> Demux/1

== system top_model/Actuator Model/Rigid Body with Momentum Actuators and energy dissipation/quat to DCM1/Subsystem ==
  In1 : Inport
  3x3 : Reshape  OutputDimensionality=Customize  OutputDimensions=[3,3]
  Demux : Demux  Outputs=3
  Gain : Gain  Gain=-1  SaturateOnIntegerOverflow=on  OutDataTypeStr=Inherit: Same as input  ParamDataTypeStr=Inherit: Same as input
  Gain1 : Gain  Gain=-1  SaturateOnIntegerOverflow=on  OutDataTypeStr=Inherit: Same as input  ParamDataTypeStr=Inherit: Same as input
  Gain2 : Gain  Gain=-1  SaturateOnIntegerOverflow=on  OutDataTypeStr=Inherit: Same as input  ParamDataTypeStr=Inherit: Same as input
  Mux : Mux  Inputs=9
  "diag 0 " : Constant  Value=0
  Out1 : Outport
  wires:
  Gain2/1 -> Mux/8
  Demux/1 -> Gain2/1, Mux/6
  Gain1/1 -> Mux/4
  Demux/2 -> Mux/7, Gain/1
  Gain/1 -> Mux/3
  Demux/3 -> Gain1/1, Mux/2
  Mux/1 -> 3x3/1
  "diag 0 "/1 -> Mux/9, Mux/5, Mux/1
  3x3/1 -> Out1/1
  In1/1 -> Demux/1

== system top_model/Attitude Determination and Desired Attitude/Attitude Determination/Generate reference vectors from Ephemeris and Magnetic Field Model/DecimalYearIncrement ==
  note: day
  clock_sec : Inport
  Add : Sum
  Constant : Constant  Value=init.year
  Constant1 : Constant  Value=init.month
  Constant2 : Constant  Value=init.day
  Constant3 : Constant  Value=init.hour
  Constant4 : Constant  Value=init.min
  Constant5 : Constant  Value=init.min
  Divide : Product  Inputs=*/
  MATLAB Function : MATLAB Function  TreatAsAtomicUnit=on
  Product2 : Product  Inputs=*/
  day2decimalYear : Constant  Value=365
  sec2day : Constant  Value=86400
  DecimalYear : Outport
  wires:
  Product2/1 -> Divide/1
  sec2day/1 -> Product2/2
  Add/1 -> DecimalYear/1
  Constant3/1 -> MATLAB Function/4(hour)
  day2decimalYear/1 -> Divide/2
  Divide/1 -> Add/1
  MATLAB Function/1(DecimalYear) -> Add/2
  Constant1/1 -> MATLAB Function/2(month)
  Constant/1 -> MATLAB Function/1(year)
  Constant4/1 -> MATLAB Function/5(minute)
  Constant5/1 -> MATLAB Function/6(second)
  clock_sec/1 -> Product2/1
  Constant2/1 -> MATLAB Function/3(day)

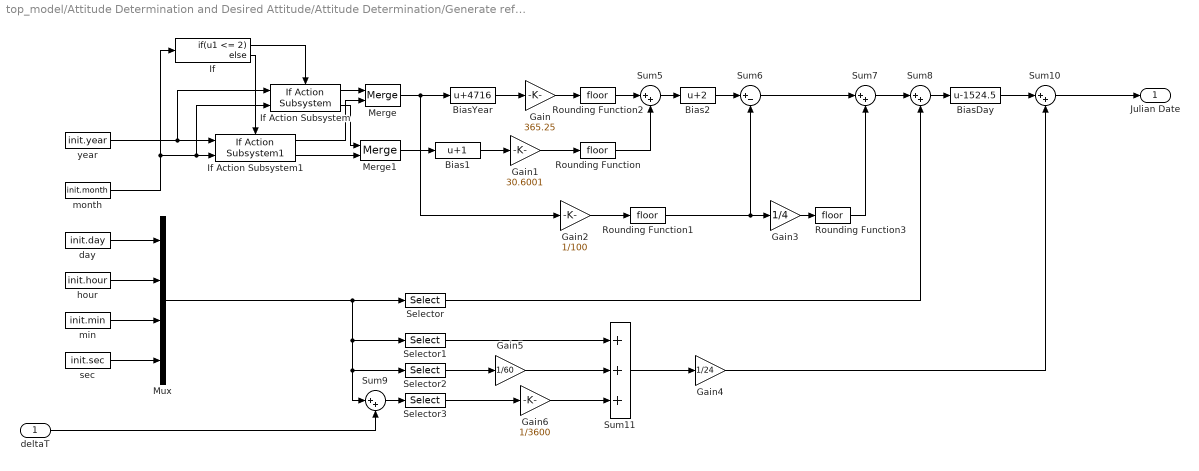
== system top_model/Attitude Determination and Desired Attitude/Attitude Determination/Generate reference vectors from Ephemeris and Magnetic Field Model/Julian Date ==
  deltaT : Inport  OutMin=0  PortDimensions=1
  Bias1 : Bias  Bias=1
  Bias2 : Bias  Bias=2
  BiasDay : Bias  Bias=-1524.5
  BiasYear : Bias  Bias=4716
  Gain : Gain  Gain=365.25
  Gain1 : Gain  Gain=30.6001
  Gain2 : Gain  Gain=1/100
  Gain3 : Gain  Gain=1/4
  Gain4 : Gain  Gain=1/24
  Gain5 : Gain  Gain=1/60
  Gain6 : Gain  Gain=1/3600
  If : If  IfExpression=u1 <= 2
  If Action Subsystem : aerolibconvert2/Julian Date Conversion/If Action Subsystem
      settings: SourceProductName=Aerospace Blockset  SourceProductBaseCode=AE
  If Action Subsystem1 : aerolibconvert2/Julian Date Conversion/If Action Subsystem1
      settings: SourceProductName=Aerospace Blockset  SourceProductBaseCode=AE
  Merge : Merge
  Merge1 : Merge
  Mux : Mux
  Rounding Function{,1..3} (4 alike) : Rounding
  Selector : Selector  InputPortWidth=4  IndexOptions=Index vector (dialog)  Indices=[1]  OutputSizes=1
  Selector1 : Selector  InputPortWidth=4  IndexOptions=Index vector (dialog)  Indices=[2]  OutputSizes=1
  Selector2 : Selector  InputPortWidth=4  IndexOptions=Index vector (dialog)  Indices=[3]  OutputSizes=1
  Selector3 : Selector  InputPortWidth=4  IndexOptions=Index vector (dialog)  Indices=[4]  OutputSizes=1
  Sum{5,7..10} (5 alike) : Sum  Inputs=|++
  Sum11 : Sum  Inputs=+++
  Sum6 : Sum  Inputs=|+-
  day : Constant  Value=init.day
  hour : Constant  Value=init.hour
  min : Constant  Value=init.min
  month : Constant  Value=init.month
  sec : Constant  Value=init.sec
  year : Constant  Value=init.year
  Julian Date : Outport
  wires:
  If Action Subsystem/1 -> Merge/1
  If/2 -> If Action Subsystem1/Action
  year/1 -> If Action Subsystem/1, If Action Subsystem1/1
  If/1 -> If Action Subsystem/Action
  If Action Subsystem/2 -> Merge1/1
  Rounding Function3/1 -> Sum7/2
  deltaT/1 -> Sum9/2
  day/1 -> Mux/1
  Merge1/1 -> Bias1/1
  Gain/1 -> Rounding Function2/1
  Gain2/1 -> Rounding Function1/1
  Merge/1 -> Gain2/1, BiasYear/1
  Selector3/1 -> Gain6/1
  Sum6/1 -> Sum7/1
  Gain5/1 -> Sum11/2
  BiasYear/1 -> Gain/1
  Selector2/1 -> Gain5/1
  Gain6/1 -> Sum11/3
  Sum11/1 -> Gain4/1
  Gain3/1 -> Rounding Function3/1
  Selector1/1 -> Sum11/1
  If Action Subsystem1/1 -> Merge/2
  Sum7/1 -> Sum8/1
  Mux/1 -> Selector1/1, Sum9/1, Selector2/1, Selector/1
  Sum10/1 -> Julian Date/1
  Selector/1 -> Sum8/2
  Bias1/1 -> Gain1/1
  sec/1 -> Mux/4
  If Action Subsystem1/2 -> Merge1/2
  Sum5/1 -> Bias2/1
  BiasDay/1 -> Sum10/1
  Gain1/1 -> Rounding Function/1
  Rounding Function1/1 -> Gain3/1, Sum6/2
  Bias2/1 -> Sum6/1
  Sum8/1 -> BiasDay/1
  Rounding Function2/1 -> Sum5/1
  Rounding Function/1 -> Sum5/2
  month/1 -> If Action Subsystem/2, If Action Subsystem1/2, If/1
  min/1 -> Mux/3
  hour/1 -> Mux/2
  Gain4/1 -> Sum10/2
  Sum9/1 -> Selector3/1

== system top_model/Attitude Determination and Desired Attitude/Position and Velocity to Desired Attitude in Quat/CreateDCM_be/normalize ==
  r : Inport
  Dot Product : DotProduct  InputSameDT=on  OutDataTypeStr=Inherit: Inherit via internal rule
  Math Function : Math  Operator=sqrt  SaturateOnIntegerOverflow=on
  Product : Product  Inputs=*/  SaturateOnIntegerOverflow=on  InputSameDT=on  OutDataTypeStr=Inherit: Same as first input
  r_hat : Outport
  wires:
  r/1 -> Dot Product/1, Dot Product/2, Product/1
  Dot Product/1 -> Math Function/1
  Math Function/1 -> Product/2
  Product/1 -> r_hat/1

== system top_model/Attitude Determination and Desired Attitude/Position and Velocity to Desired Attitude in Quat/CreateDCM_be/normalize2 ==
  v : Inport
  Dot Product : DotProduct  InputSameDT=on  OutDataTypeStr=Inherit: Inherit via internal rule
  Math Function : Math  Operator=sqrt  SaturateOnIntegerOverflow=on
  Product : Product  Inputs=*/  SaturateOnIntegerOverflow=on  InputSameDT=on  OutDataTypeStr=Inherit: Same as first input
  v_hat : Outport
  wires:
  v/1 -> Dot Product/1, Dot Product/2, Product/1
  Dot Product/1 -> Math Function/1
  Math Function/1 -> Product/2
  Product/1 -> v_hat/1

== system top_model/Attitude Determination and Desired Attitude/Position and Velocity to Desired Attitude in Quat/quat to DCM/Subsystem ==
  In1 : Inport
  3x3 : Reshape  OutputDimensionality=Customize  OutputDimensions=[3,3]
  Demux : Demux  Outputs=3
  Gain : Gain  Gain=-1  SaturateOnIntegerOverflow=on  OutDataTypeStr=Inherit: Same as input  ParamDataTypeStr=Inherit: Same as input
  Gain1 : Gain  Gain=-1  SaturateOnIntegerOverflow=on  OutDataTypeStr=Inherit: Same as input  ParamDataTypeStr=Inherit: Same as input
  Gain2 : Gain  Gain=-1  SaturateOnIntegerOverflow=on  OutDataTypeStr=Inherit: Same as input  ParamDataTypeStr=Inherit: Same as input
  Mux : Mux  Inputs=9
  "diag 0 " : Constant  Value=0
  Out1 : Outport
  wires:
  Gain2/1 -> Mux/8
  Demux/1 -> Gain2/1, Mux/6
  Gain1/1 -> Mux/4
  Demux/2 -> Mux/7, Gain/1
  Gain/1 -> Mux/3
  Demux/3 -> Gain1/1, Mux/2
  Mux/1 -> 3x3/1
  "diag 0 "/1 -> Mux/9, Mux/5, Mux/1
  3x3/1 -> Out1/1
  In1/1 -> Demux/1

== system top_model/Controller/Free Rigid Body with Momentum Actuators2/Quaternion Integration/q_normalize ==
  q_in : Inport  PortDimensions=4
  Dot Product : DotProduct  InputSameDT=on  OutDataTypeStr=Inherit: Inherit via internal rule
  Math Function : Math  Operator=sqrt  SaturateOnIntegerOverflow=on
  Product : Product  Inputs=*/  SaturateOnIntegerOverflow=on  InputSameDT=on  OutDataTypeStr=Inherit: Same as first input
  q_out : Outport
  wires:
  q_in/1 -> Dot Product/1, Dot Product/2, Product/1
  Dot Product/1 -> Math Function/1
  Math Function/1 -> Product/2
  Product/1 -> q_out/1

== system top_model/Controller/Free Rigid Body with Momentum Actuators2/Quaternion Integration/qderiv ==
  w : Inport
  q : Inport  Port=2
  Mux : Mux  Inputs=2
  Mux1 : Mux
  qd1 : Fcn  Expr=(u(7)*u(1)-u(6)*u(2)+u(5)*u(3))/2
  qd2 : Fcn  Expr=(u(6)*u(1)+u(7)*u(2)-u(4)*u(3))/2
  qd3 : Fcn  Expr=(-u(5)*u(1)+u(4)*u(2)+u(7)*u(3))/2
  qd4 : Fcn  Expr=(-u(4)*u(1)-u(5)*u(2)-u(6)*u(3))/2
  qd : Outport
  wires:
  w/1 -> Mux/1
  q/1 -> Mux/2
  Mux/1 -> qd3/1, qd4/1, qd1/1, qd2/1
  qd1/1 -> Mux1/1
  qd2/1 -> Mux1/2
  qd3/1 -> Mux1/3
  qd4/1 -> Mux1/4
  Mux1/1 -> qd/1

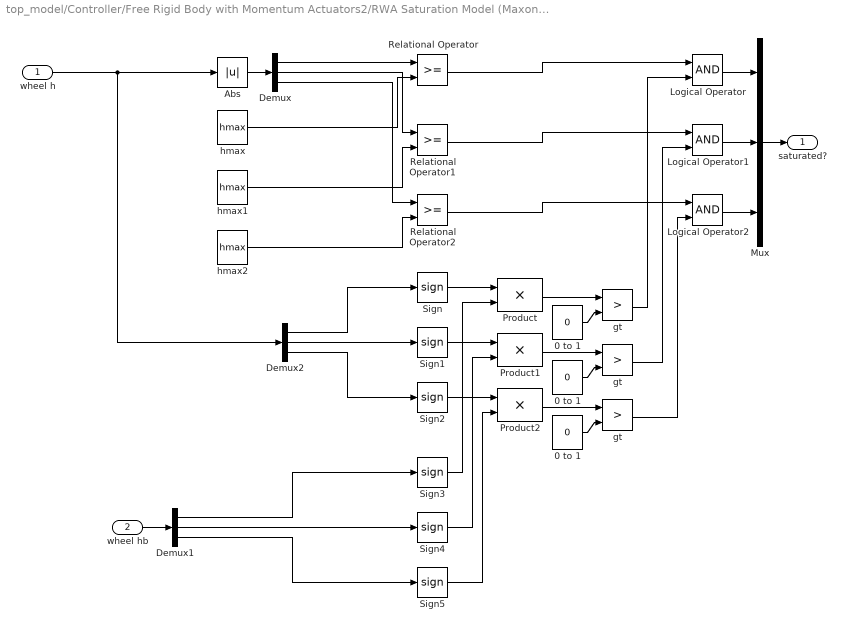
== system top_model/Controller/Free Rigid Body with Momentum Actuators2/RWA Saturation Model (Maxon EC 32 Flat 15W 24V)/max rate check ==
  wheel h : Inport
  wheel hb : Inport  Port=2
  0 to 1 : Constant  Value=0  VectorParams1D=off
  "0 to 1 " : Constant  Value=0  VectorParams1D=off
  "0 to 1  " : Constant  Value=0  VectorParams1D=off
  Abs : Abs  SaturateOnIntegerOverflow=on
  Demux : Demux  Outputs=3
  Demux1 : Demux  Outputs=3
  Demux2 : Demux  Outputs=3
  Logical Operator : Logic
  Logical Operator1 : Logic
  Logical Operator2 : Logic
  Mux : Mux  Inputs=3
  Product : Product  SaturateOnIntegerOverflow=on  InputSameDT=on  OutDataTypeStr=Inherit: Same as first input
  Product1 : Product  SaturateOnIntegerOverflow=on  InputSameDT=on  OutDataTypeStr=Inherit: Same as first input
  Product2 : Product  SaturateOnIntegerOverflow=on  InputSameDT=on  OutDataTypeStr=Inherit: Same as first input
  Relational Operator : RelationalOperator  RndMeth=Nearest  InputSameDT=on
  Relational Operator1 : RelationalOperator  RndMeth=Nearest  InputSameDT=on
  Relational Operator2 : RelationalOperator  RndMeth=Nearest  InputSameDT=on
  Sign{,1..5} (6 alike) : Signum
  gt : RelationalOperator  Operator=>  RndMeth=Nearest  InputSameDT=on
  "gt " : RelationalOperator  Operator=>  RndMeth=Nearest  InputSameDT=on
  "gt  " : RelationalOperator  Operator=>  RndMeth=Nearest  InputSameDT=on
  hmax : Constant  Value=hmax  VectorParams1D=off
  hmax1 : Constant  Value=hmax  VectorParams1D=off
  hmax2 : Constant  Value=hmax  VectorParams1D=off
  saturated? : Outport
  wires:
  Abs/1 -> Demux/1
  Demux/1 -> Relational Operator/1
  Demux/2 -> Relational Operator1/1
  Demux/3 -> Relational Operator2/1
  hmax/1 -> Relational Operator/2
  hmax1/1 -> Relational Operator1/2
  hmax2/1 -> Relational Operator2/2
  wheel h/1 -> Abs/1, Demux2/1
  Mux/1 -> saturated?/1
  wheel hb/1 -> Demux1/1
  Demux1/1 -> Sign3/1
  Demux1/2 -> Sign4/1
  Demux1/3 -> Sign5/1
  Sign/1 -> Product/1
  Sign3/1 -> Product/2
  Sign1/1 -> Product1/1
  Sign4/1 -> Product1/2
  Sign2/1 -> Product2/1
  Sign5/1 -> Product2/2
  0 to 1/1 -> gt/2
  Product/1 -> gt/1
  "0 to 1 "/1 -> "gt "/2
  Product1/1 -> "gt "/1
  "0 to 1  "/1 -> "gt  "/2
  Product2/1 -> "gt  "/1
  Logical Operator/1 -> Mux/1
  Logical Operator1/1 -> Mux/2
  Logical Operator2/1 -> Mux/3
  Relational Operator/1 -> Logical Operator/1
  Relational Operator1/1 -> Logical Operator1/1
  Relational Operator2/1 -> Logical Operator2/1
  gt/1 -> Logical Operator/2
  "gt "/1 -> Logical Operator1/2
  "gt  "/1 -> Logical Operator2/2
  Demux2/1 -> Sign/1
  Demux2/2 -> Sign1/1
  Demux2/3 -> Sign2/1

== system top_model/Controller/Free Rigid Body with Momentum Actuators2/compute attitude error/quat_multiply (relative quat) ==
  q_bc : Inport
  q_ab : Inport  Port=2
  Mux : Mux  Inputs=2
  Mux1 : Mux
  qerr1 : Fcn  Expr=u(4)*u(5)+u(3)*u(6)-u(2)*u(7)+u(1)*u(8)
  qerr2 : Fcn  Expr=-u(3)*u(5)+u(4)*u(6)+u(1)*u(7)+u(2)*u(8)
  qerr3 : Fcn  Expr=u(2)*u(5)-u(1)*u(6)+u(4)*u(7)+u(3)*u(8)
  qerr4 : Fcn  Expr=-u(1)*u(5)-u(2)*u(6)-u(3)*u(7)+u(4)*u(8)
  q_ac : Outport
  wires:
  Mux1/1 -> q_ac/1
  qerr4/1 -> Mux1/4
  qerr3/1 -> Mux1/3
  qerr2/1 -> Mux1/2
  qerr1/1 -> Mux1/1
  Mux/1 -> qerr4/1, qerr3/1, qerr2/1, qerr1/1
  q_ab/1 -> Mux/2
  q_bc/1 -> Mux/1

== system top_model/Controller/Normal Mode Control System/compute attitude error/quat_multiply (relative quat) ==
  q_bc : Inport
  q_ab : Inport  Port=2
  Mux : Mux  Inputs=2
  Mux1 : Mux
  qerr1 : Fcn  Expr=u(4)*u(5)+u(3)*u(6)-u(2)*u(7)+u(1)*u(8)
  qerr2 : Fcn  Expr=-u(3)*u(5)+u(4)*u(6)+u(1)*u(7)+u(2)*u(8)
  qerr3 : Fcn  Expr=u(2)*u(5)-u(1)*u(6)+u(4)*u(7)+u(3)*u(8)
  qerr4 : Fcn  Expr=-u(1)*u(5)-u(2)*u(6)-u(3)*u(7)+u(4)*u(8)
  q_ac : Outport
  wires:
  Mux1/1 -> q_ac/1
  qerr4/1 -> Mux1/4
  qerr3/1 -> Mux1/3
  qerr2/1 -> Mux1/2
  qerr1/1 -> Mux1/1
  Mux/1 -> qerr4/1, qerr3/1, qerr2/1, qerr1/1
  q_ab/1 -> Mux/2
  q_bc/1 -> Mux/1

== system top_model/Controller/Normal Mode Control System/compute attitude error/quat_multiply (relative quat)1 ==
  q_bc : Inport
  q_ab : Inport  Port=2
  Mux : Mux  Inputs=2
  Mux1 : Mux
  qerr1 : Fcn  Expr=u(4)*u(5)+u(3)*u(6)-u(2)*u(7)+u(1)*u(8)
  qerr2 : Fcn  Expr=-u(3)*u(5)+u(4)*u(6)+u(1)*u(7)+u(2)*u(8)
  qerr3 : Fcn  Expr=u(2)*u(5)-u(1)*u(6)+u(4)*u(7)+u(3)*u(8)
  qerr4 : Fcn  Expr=-u(1)*u(5)-u(2)*u(6)-u(3)*u(7)+u(4)*u(8)
  q_ac : Outport
  wires:
  Mux1/1 -> q_ac/1
  qerr4/1 -> Mux1/4
  qerr3/1 -> Mux1/3
  qerr2/1 -> Mux1/2
  qerr1/1 -> Mux1/1
  Mux/1 -> qerr4/1, qerr3/1, qerr2/1, qerr1/1
  q_ab/1 -> Mux/2
  q_bc/1 -> Mux/1

== system top_model/GNC/Follower Maneuver/Optimal Latitude Calc/Enabled Subsystem ==
  r : Inport
  v : Inport  Port=2
  x_tgt : Inport  Port=3
  x_f : Inport  Port=4
  K : Inport  Port=5
  L : Inport  Port=6
  "muE " : Inport  Port=7
  Enable : EnablePort
  MATLAB Function : MATLAB Function  TreatAsAtomicUnit=on
  dV_opt : Outport
  long_opt : Outport  Port=2
  pos_opt : Outport  Port=3
  wires:
  r/1 -> MATLAB Function/1(r)
  v/1 -> MATLAB Function/2(v)
  "muE "/1 -> MATLAB Function/7(muE)
  x_tgt/1 -> MATLAB Function/3(x_t)
  x_f/1 -> MATLAB Function/4(x)
  K/1 -> MATLAB Function/5(K)
  L/1 -> MATLAB Function/6(L)
  MATLAB Function/3(long_opt) -> long_opt/1
  MATLAB Function/1(dV_opt) -> dV_opt/1
  MATLAB Function/2(pos_opt) -> pos_opt/1

== matlab function top_model/FWR_Plant/Atmospheric drag ==
  data: velocity input; drag output
function drag = fcn(velocity)
V= norm(velocity);    % 
A= 0.01*0.01;   % 10cm x 10cm
Cd= 0.82;       % for long square cylinder
drag = Cd * A * .5 * 1e-8 * V * -velocity;
